simulink model "Supercap_Thermo_Electrical_Cell_Simulation_Model"  (R2024b)
settings: Solver=VariableStepAuto  StartTime=0.0  StopTime=Sim_TimeEnd_s
undefined symbols (not defined in the file): C, Cell_CapRated_F, Cell_HeatCapa_JpK, Cell_LowerSOCLimit_pc, Cell_LowerVoltageLimit_V, Cell_ResESR10ms_Ohm, Cell_ResESR1s_Ohm, Cell_RthToCooling_KpW, Cell_RthToEnvironment_KpW, Cell_TempInit_degC, Cell_UpperSOCLimit_pc, Cell_UpperVoltageLimit_V, Cell_VoltRated_V, Cell_VoltStart_V, Cooling_Temp_degC, Environment_Temp_degC, ESR, Sim_SocInit_pc, Sim_SOH_PU, Sim_TimeStep_s, Switch_CoolingONOFF, Switch_CurrentOrPower, Switch_DeratingONOFF_NN
libraries: simulink x11, slpidlib x1
settings Model: Creator=ludovico.barro  LastModifiedBy=francesco.bazzani
settings ModelReferenceCC: EnableRefExpFcnMdlSchedulingChecks=on
settings RTWCC: GPUComputeCapability=3.5

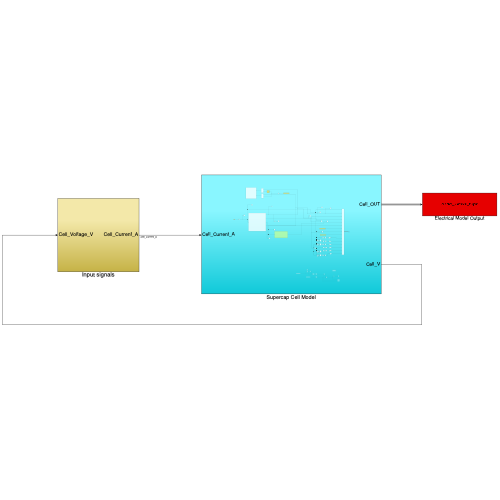
[thumbnail: Simulink's stored preview of the top-level diagram]
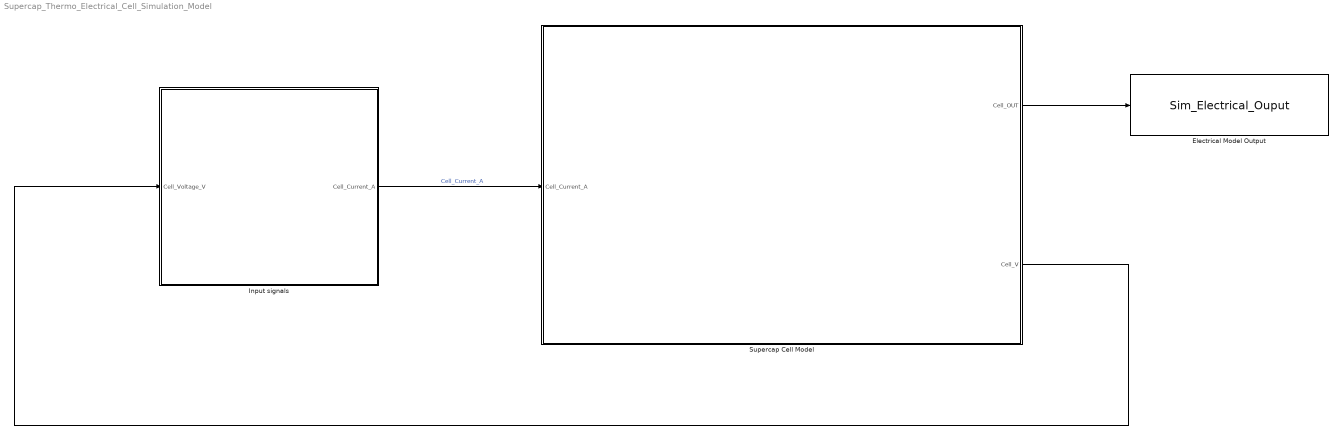
== system Supercap_Thermo_Electrical_Cell_Simulation_Model ==
  Electrical Model Output : ToWorkspace  VariableName=Sim_Electrical_Ouput  SaveFormat=Timeseries  SampleTime=Sim_TimeStep_s
  Input signals : Subsystem
  Supercap Cell Model : Subsystem
  wires:
  Supercap Cell Model/1(Cell_OUT) -> Electrical Model Output/1
  Input signals/1(Cell_Current_A) -> Supercap Cell Model/1(Cell_Current_A)  "Cell_Current_A"
  Supercap Cell Model/2(Cell_V) -> Input signals/1(Cell_Voltage_V)

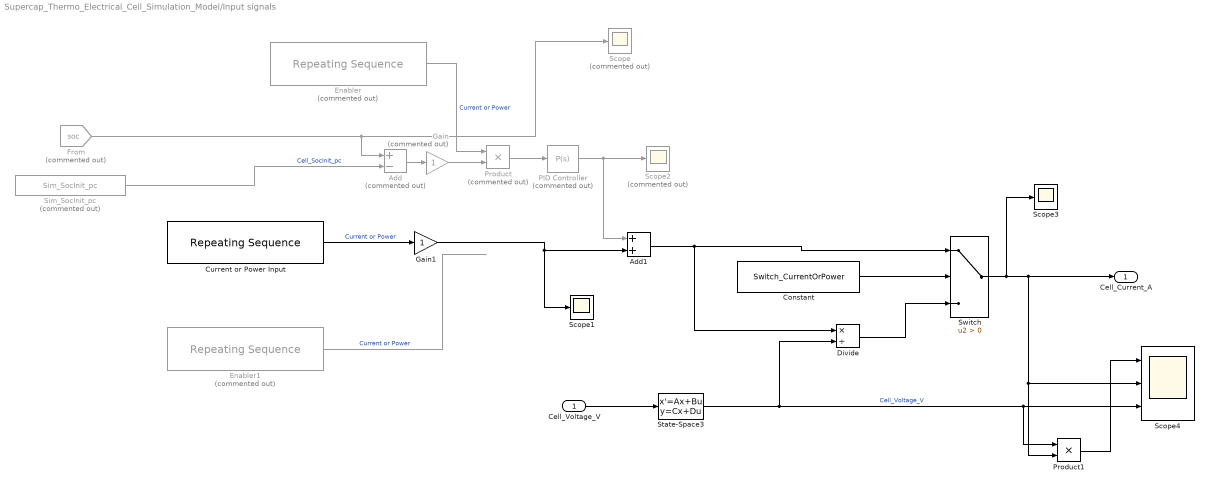
== system Supercap_Thermo_Electrical_Cell_Simulation_Model/Input signals ==
  Cell_Voltage_V : Inport
  Add : Sum  Commented=on  Inputs=+-
  Add1 : Sum
  Constant : Constant  Value=Switch_CurrentOrPower
  Current or Power Input : simulink/Sources/Repeating Sequence  rep_seq_t=Cell_LoadInputTime_s  rep_seq_y=Cell_LoadInputCurrOrPower_AW
  Divide : Product  Inputs=*/
  Enabler : simulink/Sources/Repeating Sequence  Commented=on  rep_seq_t=[0, 60,60.1, 20*60, 20*60+0.1]  rep_seq_y=[0,0,1,1,0]
  Enabler1 : simulink/Sources/Repeating Sequence  Commented=on  rep_seq_t=[0, 60,60.1, 20*60, 20*60+0.1]  rep_seq_y=[1,1,0,0,1]
  From : From  Commented=on  GotoTag=soc  TagVisibility=global
  Gain : Gain  Commented=on
  Gain1 : Gain
  PID Controller : slpidlib/PID Controller  Commented=on  Controller=P  Form=Parallel  TimeDomain=Continuous-time  UseExternalTs=off  SampleTime=-1  IntegratorMethod=Forward Euler  FilterMethod=Forward Euler  ControllerParametersSource=internal  P=1000  I=1  UseKiTs=off  D=0  UseExternalDerivativeSource=off  N=100  UseFilter=on  TunerSelectOption=Transfer Function Based (PID Tuner App)  InitialConditionSource=internal  InitialConditionForIntegrator=0  InitialConditionForFilter=0  DifferentiatorICPrevScaledInput=0  ExternalReset=none  TrackingMode=off  Kt=1  LimitOutput=on  SatLimitsSource=internal  UpperSaturationLimit=10  LowerSaturationLimit=-10  LinearizeAsGain=on  AntiWindupMode=none  Kb=1  LimitIntegrator=off  UpperIntegratorSaturationLimit=inf  LowerIntegratorSaturationLimit=-inf  POutMin=[]  POutMax=[]  IOutMin=[]  IOutMax=[]  DOutMin=[]  DOutMax=[]  NOutMin=[]  NOutMax=[]  SumOutMin=[]  SumOutMax=[]  SaturationOutMin=[]  SaturationOutMax=[]  PParamMin=[]  PParamMax=[]  IParamMin=[]  IParamMax=[]  DParamMin=[]  DParamMax=[]  NParamMin=[]  NParamMax=[]  KbParamMin=[]  KbParamMax=[]  KtParamMin=[]  KtParamMax=[]  KbOutMin=[]  KbOutMax=[]  KtOutMin=[]  KtOutMax=[]  IntegratorOutMin=[]  IntegratorOutMax=[]  FilterOutMin=[]  FilterOutMax=[]  SumI1OutMin=[]  SumI1OutMax=[]  SumI2OutMin=[]  SumI2OutMax=[]  SumI3OutMin=[]  SumI3OutMax=[]  SumI4OutMin=[]  SumI4OutMax=[]  SumDOutMin=[]  SumDOutMax=[]  DifferentiatorOutMin=[]  DifferentiatorOutMax=[]  FilterDiffOutCoefMin=[]  FilterDiffOutCoefMax=[]  ReciprocalOutMin=[]  ReciprocalOutMax=[]  SumDenOutMin=[]  SumDenOutMax=[]  SumNumOutMin=[]  SumNumOutMax=[]  DivideOutMin=[]  DivideOutMax=[]  UdiffTsProdOutMin=[]  UdiffTsProdOutMax=[]  NTsProdOutMin=[]  NTsProdOutMax=[]  UintegralTsProdOutMin=[]  UintegralTsProdOutMax=[]  UngainTsProdOutMin=[]  UngainTsProdOutMax=[]  ClampingZeroOutDataTypeStr=Inherit: Inherit via back propagation  ClampingZeroOutMin=[]  ClampingZeroOutMax=[]  FilterDenConstantOutDataTypeStr=Inherit: Inherit via back propagation  FilterDenConstantOutMin=[]  FilterDenConstantOutMax=[]  PCopyOutDataTypeStr=Inherit: Inherit via back propagation  PCopyOutMin=[]  PCopyOutMax=[]  NCopyOutDataTypeStr=Inherit: Inherit via back propagation  NCopyOutMin=[]  NCopyOutMax=[]  IntegratorContinuousStateAttributes=''  IntegratorStateMustResolveToSignalObject=off  IntegratorRTWStateStorageClass=Auto  FilterContinuousStateAttributes=''  FilterStateMustResolveToSignalObject=off  FilterRTWStateStorageClass=Auto  ParallelPVariant=InternalParameters  IdealPVariant=Disabled  IVariant=Disabled  DVariant=Disabled  IntegratorVariant=Disabled  SatVariant=Enabled  AWVariant=Disabled  PCopyVariant=Disabled  TRVariant=Disabled  FdbkBlocksVariant=Forward  IdealPFdbkVariant=Disabled  SatFdbkVariant=Disabled  DerivativeFilterVariant=Disabled  NVariant=Disabled  NCopyVariant=Disabled_SignalSpec  FilterICVariant=Disabled  IntegratorICVariant=Disabled  ExternalResetVariant=Disabled  TRSumVariant=Passthrough  SumFdbkVariant=Disabled  SumVariant=Passthrough_P  TsampFilterVariant=InternalTs  TsampNgainVariant=Passthrough  TsampIntegralVariant=Disabled_SignalSpec  ExternalSaturationOutDataTypeStr=Inherit: Same as second input  DerivativeSourceVariant=Disabled  PreIntVariant=InternalPreInt
  Product : Product  Commented=on
  Product1 : Product
  Scope : Scope  Commented=on
  Scope1 : Scope
  Scope2 : Scope  Commented=on
  Scope3 : Scope
  Scope4 : Scope  NumInputPorts=3
  Sim_SocInit_pc : Constant  Commented=on  Value=Sim_SocInit_pc
  State-Space3 : StateSpace  A=-1/1e-6  B=1/1e-6  D=0  InitialCondition=Cell_VoltStart_V
  Switch : Switch  Criteria=u2 > Threshold  SaturateOnIntegerOverflow=off  InputSameDT=off
  Cell_Current_A : Outport
  wires:
  Constant/1 -> Switch/2
  Switch/1 -> Scope3/1, Scope4/2, Product1/2, Cell_Current_A/1
  Cell_Voltage_V/1 -> State-Space3/1
  State-Space3/1 -> Product1/1, Scope4/3, Divide/2  "Cell_Voltage_V"
  Divide/1 -> Switch/3
  Sim_SocInit_pc/1 -> Add/2  "Cell_SocInit_pc"
  From/1 -> Add/1, Scope/1
  Add/1 -> Gain/1
  Product/1 -> PID Controller/1
  Enabler/1 -> Product/1  "Current or Power"
  PID Controller/1 -> Scope2/1, Add1/1
  Add1/1 -> Divide/1, Switch/1
  Current or Power Input/1 -> Gain1/1  "Current or Power"
  Gain1/1 -> Scope1/1, Add1/2
  Enabler1/1 -> ?  "Current or Power"
  Gain/1 -> Product/2
  Product1/1 -> Scope4/1

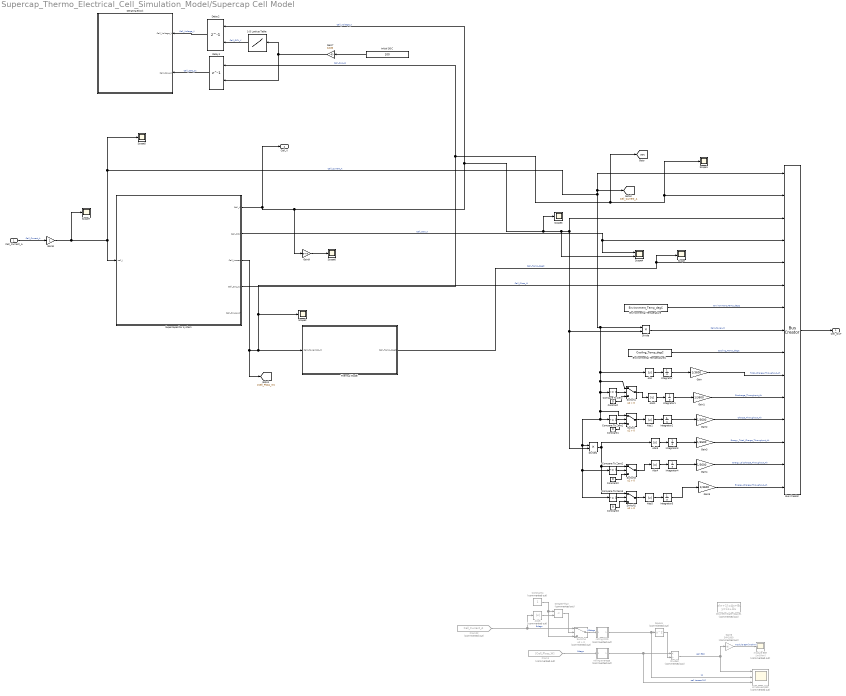
== system Supercap_Thermo_Electrical_Cell_Simulation_Model/Supercap Cell Model ==
  Cell_Current_A : Inport
  1-D Lookup Table : Lookup_n-D  NumberOfTableDimensions=1  BreakpointsForDimension1=linspace(0,1,1000)  Table=linspace(0,1,1000).^(1/2)*3  InternalRulePriority=Speed  RndMeth=Simplest
  Abs{,1..5} (6 alike) : Abs  SaturateOnIntegerOverflow=off
  Abs6 : Abs  Commented=on  SaturateOnIntegerOverflow=off
  Bus Creator : BusCreator  Inputs=15
  Compare To Zero : simulink/Logic and Bit Operations/Compare To Zero  relop=<=  OutDataTypeStr=boolean
  Compare To Zero1 : simulink/Logic and Bit Operations/Compare To Zero  relop=>=  OutDataTypeStr=boolean
  Compare To Zero2 : simulink/Logic and Bit Operations/Compare To Zero  relop=<=  OutDataTypeStr=boolean
  Compare To Zero3 : simulink/Logic and Bit Operations/Compare To Zero  relop=>=  OutDataTypeStr=boolean
  Constant{,1..3} (4 alike) : Constant  Value=0
  Constant4 : Constant  Commented=on
  Delay1 : Delay  DelayLength=1  InitialConditionSource=Input port
      settings: InputPortMap=u0,p4
  Delay2 : Delay  DelayLength=1  InitialConditionSource=Input port
      settings: InputPortMap=u0,p4
  Derating Block : Subsystem
  Discrete State-Space1 : DiscreteStateSpace  Commented=on  A=-1/(1e-6)  B=1/(1e-6)  D=0  SampleTime=-1
  Divide : Product  Inputs=**
  Divide1 : Product  Inputs=**
  Divide2 : Product  Commented=on  Inputs=*/
  Environmental Temperature : Constant  Value=Environment_Temp_degC
  Environmental Temperature1 : Constant  Value=Cooling_Temp_degC
  From1 : From  Commented=on  GotoTag=Cell_Ploss_W
  From22 : From  Commented=on  GotoTag=Cell_Current_A  TagVisibility=global
  Gain{,1..5} (6 alike) : Gain  Gain=1/3600
  Gain6 : Gain  Commented=on  Gain=54*1000
  Gain7 : Gain  Gain=1/100
  Gain8 : Gain
  Gain9 : Gain  Gain=54*9
  GreaterThan : RelationalOperator  Commented=on  Operator=<  OutDataTypeStr=boolean  RndMeth=Simplest  InputSameDT=off
  Initial SOC : Constant  Value=100
  Integrator{,1..5} (6 alike) : Integrator
  Scope{,1..3,5..7} (7 alike) : Scope
  Scope4 : Scope  NumInputPorts=2
  Square : Math  Commented=on  Operator=square
  Supercapacitor system : Subsystem  mask{Cell_ResESR10ms_Ohm=Cell_ResESR10ms_Ohm, Cell_ResESR1s_Ohm=Cell_ResESR1s_Ohm, Cell_CapRated_F=Cell_CapRated_F, Cell_VoltRated_V=Cell_VoltRated_V, Cell_SoCInit_PU=Sim_SocInit_pc, Cell_SOH_PU=Sim_SOH_PU, cell_count=54, add_Res=1.12, bridge_Res=0.8}
      mask prompts: Cell_ResESR10ms_Ohm "Rated 10ms ESR [Ohm]"; Cell_ResESR1s_Ohm "Rated 1s ESR [Ohm]"; Cell_CapRated_F "Rated Capacitance [F]"; Cell_VoltRated_V "Rated V [V]"; Cell_SoCInit_PU "SoC [PU]"; Cell_SOH_PU "SoH [PU]"; cell_count "cells per module"; add_Res "Additional module R"; bridge_Res "Bridge R"
      mask DialogControl Container6 Prompt: Cell
      mask DialogControl Container4 Prompt: Module
      mask Display: image('Skeleton-SCX5000-300x300.jpg');
  Switch{,1..3} (4 alike) : Switch  Criteria=u2 > Threshold  SaturateOnIntegerOverflow=off  InputSameDT=off
  Switch4 : Switch  Commented=on  Criteria=u2 > Threshold  SaturateOnIntegerOverflow=off  InputSameDT=off
  Thermal Model : Subsystem
      mask Display: image('fluid_flow.png'); % Use "Edit Image" on toolstrip to change.
  Windowed ESR : Scope  Commented=on  NumInputPorts=3
  module ESR [mOhm] : Scope  Commented=on
  rolling RMS : Subsystem  Commented=on  mask{t_window=60}
      mask prompts: t_window "window time [s]"
  rolling average : Subsystem  Commented=on  mask{t_window=60}
      mask prompts: t_window "window time [s]"
  Cell_OUT : Outport
  Cell_V : Outport  Port=2
  tag scope: Cell_Current_A=global, soc=global
  wires:
  Thermal Model/1(Cell_Temp_degC) -> Scope/1, Bus Creator/5  "Cell_Temp_degC"
  Supercapacitor system/3(Cell_Losses) -> Thermal Model/1(Cell_Powerloss_W), Scope2/1, Bus Creator/6, [Cell_Ploss_W]  "Cell_Ploss_W"
  Supercapacitor system/4(Cell_Soc_pu) -> Delay1/1, [soc], Scope1/1, Bus Creator/2  "Cell_Soc_pc"
  Environmental Temperature/1 -> Bus Creator/7  "Environment_Temp_degC"
  Supercapacitor system/1(Cell_V) -> Cell_V/1, Gain9/1, Delay2/1, Scope3/1, Scope4/2, Bus Creator/3, Divide1/2, Divide/2  "Cell_Voltage_V"
  Supercapacitor system/2(Cell_OCV) -> Scope4/1, Bus Creator/4  "Cell_OCV_V"
  Bus Creator/1 -> Cell_OUT/1
  Divide/1 -> Bus Creator/8  "Cell_Power_W"
  Environmental Temperature1/1 -> Bus Creator/9  "Cooling_Temp_degC"
  Delay1/1 -> Derating Block/2(Cell_Soc_pc)  "Cell_SOC_pc"
  1-D Lookup Table/1 -> Delay2/2  "Cell_OCV_V"
  Delay2/1 -> Derating Block/1(Cell_Voltage_V)  "Cell_Voltage_V"
  Initial SOC/1 -> Gain7/1
  Integrator/1 -> Gain/1
  Abs/1 -> Integrator/1
  Gain/1 -> Bus Creator/10  "Total_Charge_Throughput_Ah"
  Gain1/1 -> Bus Creator/11  "Discharge_Throughput_Ah"
  Switch1/1 -> Abs1/1
  Integrator1/1 -> Gain1/1
  Integrator2/1 -> Gain2/1
  Switch/1 -> Abs2/1
  Gain2/1 -> Bus Creator/12  "Charge_Throughput_Ah"
  Abs1/1 -> Integrator1/1
  Abs2/1 -> Integrator2/1
  Compare To Zero/1 -> Switch1/2
  Constant/1 -> Switch1/3
  Constant1/1 -> Switch/3
  Compare To Zero1/1 -> Switch/2
  Compare To Zero3/1 -> Switch2/2
  Constant3/1 -> Switch2/3
  Constant2/1 -> Switch3/3
  Compare To Zero2/1 -> Switch3/2
  Abs5/1 -> Integrator5/1
  Abs4/1 -> Integrator4/1
  Gain5/1 -> Bus Creator/15  "Energy_Charge_Throughput_Ah"
  Switch2/1 -> Abs5/1
  Integrator5/1 -> Gain5/1
  Cell_Current_A/1 -> Gain8/1  "Cell_Current_A"
  Integrator4/1 -> Gain4/1
  Switch3/1 -> Abs4/1
  Gain4/1 -> Bus Creator/14  "Energy_Discharge_Throughput_Ah"
  Gain3/1 -> Bus Creator/13  "Energy_Total_Charge_Throughput_Ah"
  Abs3/1 -> Integrator3/1
  Integrator3/1 -> Gain3/1
  Divide1/1 -> Abs3/1, Switch2/1, Switch3/1
  Constant4/1 -> Switch4/3, GreaterThan/1
  rolling average/1(Out1) -> Divide2/1, Windowed ESR/3  "cell Losses [W]"
  Switch4/1 -> rolling RMS/1(In1)  "55degc"
  Gain6/1 -> module ESR [mOhm]/1  "module ESR [mOhm]"
  Abs6/1 -> GreaterThan/2
  Square/1 -> Divide2/2
  Divide2/1 -> Windowed ESR/1, Gain6/1  "cell ESR"
  rolling RMS/1(Out1) -> Windowed ESR/2, Square/1  "1s"
  From22/1 -> Switch4/1, Abs6/1  "5degc"
  GreaterThan/1 -> Switch4/2
  From1/1 -> rolling average/1(In1)  "5degc"
  Gain7/1 -> Delay1/2, 1-D Lookup Table/1
  Gain8/1 -> Scope7/1, Scope5/1, [Cell_Current_A], Bus Creator/1, Compare To Zero1/1, Compare To Zero3/1, Compare To Zero2/1, Divide1/1, Switch/1, Compare To Zero/1, Switch1/1, Abs/1, Divide/1, Supercapacitor system/1(cell_I)  "Cell_Current_A"
  Gain9/1 -> Scope6/1

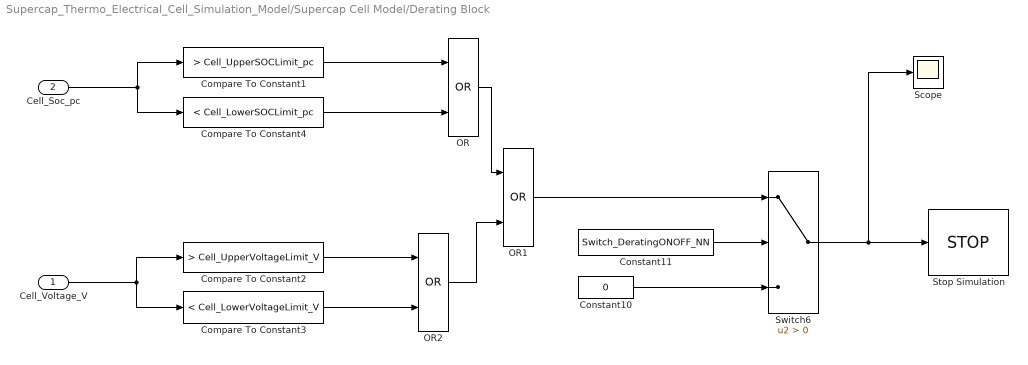
== system Supercap_Thermo_Electrical_Cell_Simulation_Model/Supercap Cell Model/Derating Block ==
  Cell_Voltage_V : Inport
  Cell_Soc_pc : Inport  Port=2
  Compare To Constant1 : simulink/Logic and Bit Operations/Compare To Constant  relop=>  const=Cell_UpperSOCLimit_pc  OutDataTypeStr=boolean
  Compare To Constant2 : simulink/Logic and Bit Operations/Compare To Constant  relop=>  const=Cell_UpperVoltageLimit_V  OutDataTypeStr=boolean
  Compare To Constant3 : simulink/Logic and Bit Operations/Compare To Constant  relop=<  const=Cell_LowerVoltageLimit_V  OutDataTypeStr=boolean
  Compare To Constant4 : simulink/Logic and Bit Operations/Compare To Constant  relop=<  const=Cell_LowerSOCLimit_pc  OutDataTypeStr=boolean
  Constant10 : Constant  Value=0
  Constant11 : Constant  Value=Switch_DeratingONOFF_NN
  OR : Logic  Operator=OR  IconShape=distinctive  AllPortsSameDT=off  OutDataTypeStr=boolean
  OR1 : Logic  Operator=OR  IconShape=distinctive  AllPortsSameDT=off  OutDataTypeStr=boolean
  OR2 : Logic  Operator=OR  IconShape=distinctive  AllPortsSameDT=off  OutDataTypeStr=boolean
  Scope : Scope
  Stop Simulation : Stop
  Switch6 : Switch  Criteria=u2 > Threshold  SaturateOnIntegerOverflow=off  InputSameDT=off
  wires:
  Cell_Soc_pc/1 -> Compare To Constant1/1, Compare To Constant4/1
  Compare To Constant4/1 -> OR/2
  Compare To Constant1/1 -> OR/1
  Cell_Voltage_V/1 -> Compare To Constant3/1, Compare To Constant2/1
  OR/1 -> OR1/1
  OR2/1 -> OR1/2
  OR1/1 -> Switch6/1
  Switch6/1 -> Scope/1, Stop Simulation/1
  Constant11/1 -> Switch6/2
  Constant10/1 -> Switch6/3
  Compare To Constant2/1 -> OR2/1
  Compare To Constant3/1 -> OR2/2

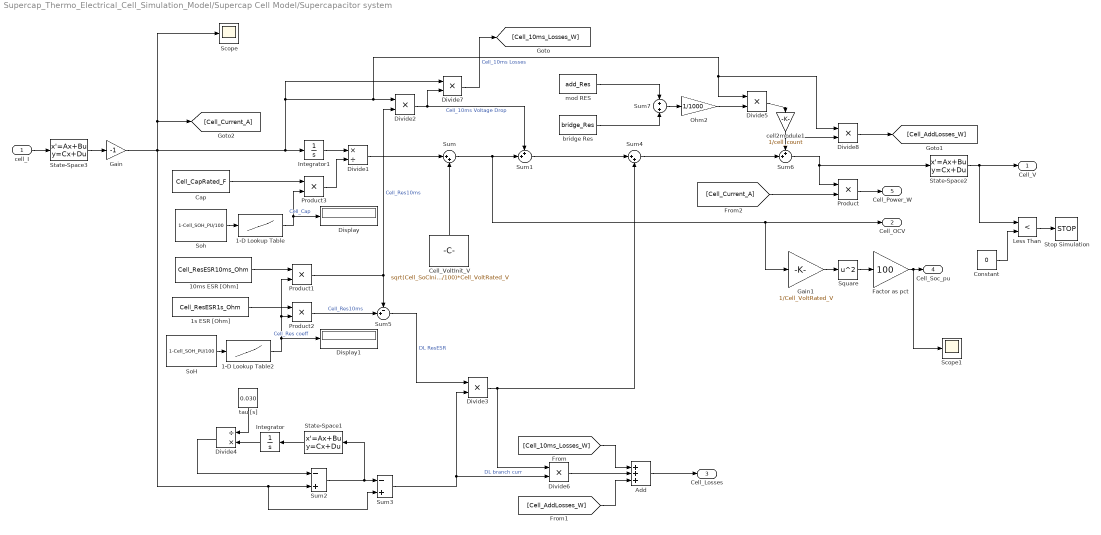
== system Supercap_Thermo_Electrical_Cell_Simulation_Model/Supercap Cell Model/Supercapacitor system ==
  cell_I : Inport
  1-D Lookup Table : Lookup_n-D  NumberOfTableDimensions=1  BreakpointsForDimension1=C(:,1)  Table=C(:,2)  InternalRulePriority=Speed  RndMeth=Simplest
  1-D Lookup Table2 : Lookup_n-D  NumberOfTableDimensions=1  BreakpointsForDimension1=ESR(:,1)  Table=ESR(:,2)  InternalRulePriority=Speed  RndMeth=Simplest
  10ms ESR [Ohm] : Constant  Value=Cell_ResESR10ms_Ohm
  1s ESR [Ohm] : Constant  Value=Cell_ResESR1s_Ohm
  Add : Sum  Inputs=+++
  Cap : Constant  Value=Cell_CapRated_F
  Cell_VoltInit_V : Constant  Value=sqrt(Cell_SoCInit_PU/100)*Cell_VoltRated_V
  Constant : Constant  Value=0
  Display : Display
  Display1 : Display
  Divide1 : Product  Inputs=*/
  Divide{2..3,5..8} (6 alike) : Product  Inputs=**
  Divide4 : Product  Inputs=/*
  Factor as pct : Gain  Gain=100
  Gain : Gain  Gain=-1
  Gain1 : Gain  Gain=1/Cell_VoltRated_V
  Integrator : Integrator
  Integrator1 : Integrator
  Less Than : RelationalOperator  Operator=<  OutDataTypeStr=boolean  RndMeth=Simplest  InputSameDT=off
  Ohm2 : Gain  Gain=1/1000
  Product{,1..3} (4 alike) : Product
  Scope : Scope
  Scope1 : Scope
  SoH : Constant  Value=1-Cell_SOH_PU/100
  Soh : Constant  Value=1-Cell_SOH_PU/100
  Square : Math  Operator=square
  State-Space1 : StateSpace  A=-1/1e-6  B=1/1e-6  D=0  InitialCondition=0
  State-Space2 : StateSpace  A=-1/1e-6  B=1/1e-6  D=0  InitialCondition=sqrt(Cell_SoCInit_PU/100)*Cell_VoltRated_V
  State-Space3 : StateSpace  A=-1/1e-6  B=1/1e-6  D=0  InitialCondition=0
  Stop Simulation : Stop
  Sum : Sum  Inputs=|++
  Sum1 : Sum  Inputs=++|
  Sum2 : Sum  Inputs=-+
  Sum3 : Sum  Inputs=-+
  Sum4 : Sum  Inputs=|++
  Sum5 : Sum  Inputs=-+|
  Sum6 : Sum  Inputs=++|
  Sum7 : Sum  Inputs=+|+
  bridge Res : Constant  Value=bridge_Res
  cell2module1 : Gain  Gain=1/cell_count
  mod RES : Constant  Value=add_Res
  tau [s] : Constant  Value=0.030
  Cell_V : Outport
  Cell_OCV : Outport  Port=2
  Cell_Losses : Outport  Port=3
  Cell_Soc_pu : Outport  Port=4
  Cell_Power_W : Outport  Port=5
  wires:
  Cell_VoltInit_V/1 -> Sum/2
  Integrator1/1 -> Divide1/1
  Product1/1 -> Sum5/1, Divide2/2  "Cell_Res10ms"
  Divide2/1 -> Divide7/2, Sum1/1  "Cell_10ms Voltage Drop"
  tau [s]/1 -> Divide4/1
  Divide3/1 -> Sum4/2, Divide6/1
  Sum1/1 -> Sum4/1
  Divide4/1 -> Sum2/1
  Divide1/1 -> Sum/1
  Sum2/1 -> Sum3/1, State-Space1/1
  Sum5/1 -> Divide3/1  "DL ResESR"
  Integrator/1 -> Divide4/2
  Sum3/1 -> Divide3/2, Divide6/2  "DL branch curr"
  cell_I/1 -> State-Space3/1
  Sum4/1 -> Sum6/2
  Sum6/1 -> Product/1, State-Space2/1
  Divide5/1 -> cell2module1/1
  mod RES/1 -> Sum7/1
  Ohm2/1 -> Divide5/2
  Sum7/1 -> Ohm2/1
  bridge Res/1 -> Sum7/2
  cell2module1/1 -> Sum6/1, Divide8/2
  Gain/1 -> Scope/1, [Cell_Current_A], Integrator1/1, Divide7/1, Divide8/1, Divide5/1, Divide2/1, Sum3/2, Sum2/2
  Divide6/1 -> Add/2
  Divide7/1 -> [Cell_10ms_Losses_W]  "Cell_10ms Losses"
  [Cell_10ms_Losses_W] -> Add/1
  Add/1 -> Cell_Losses/1
  Divide8/1 -> [Cell_AddLosses_W]
  [Cell_AddLosses_W] -> Add/3
  Gain1/1 -> Square/1
  Square/1 -> Factor as pct/1
  [Cell_Current_A] -> Product/2
  Product/1 -> Cell_Power_W/1
  Sum/1 -> Gain1/1, Cell_OCV/1, Sum1/2
  State-Space1/1 -> Integrator/1
  State-Space2/1 -> Less Than/1, Cell_V/1
  State-Space3/1 -> Gain/1
  Factor as pct/1 -> Scope1/1, Cell_Soc_pu/1
  Constant/1 -> Less Than/2
  Less Than/1 -> Stop Simulation/1
  SoH/1 -> 1-D Lookup Table2/1
  10ms ESR [Ohm]/1 -> Product1/1
  1-D Lookup Table2/1 -> Display1/1, Product2/2, Product1/2  "Cell_Res coeff"
  1s ESR [Ohm]/1 -> Product2/1
  Product2/1 -> Sum5/2  "Cell_Res10ms"
  Soh/1 -> 1-D Lookup Table/1
  1-D Lookup Table/1 -> Display/1, Product3/2  "Cell_Cap"
  Cap/1 -> Product3/1
  Product3/1 -> Divide1/2

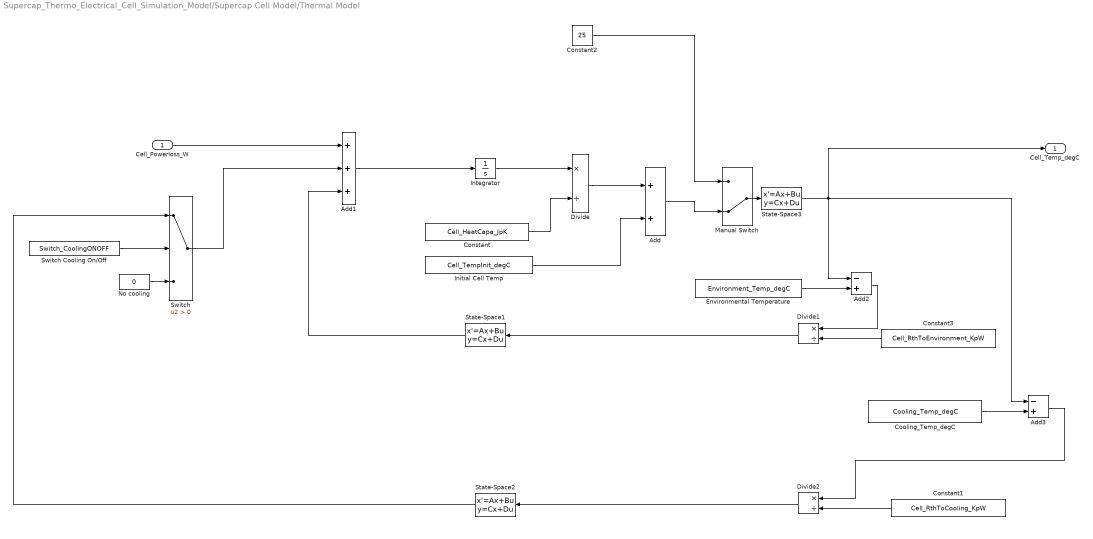
== system Supercap_Thermo_Electrical_Cell_Simulation_Model/Supercap Cell Model/Thermal Model ==
  Cell_Powerloss_W : Inport
  Add : Sum
  Add1 : Sum  Inputs=+++
  Add2 : Sum  Inputs=-+
  Add3 : Sum  Inputs=-+
  Constant : Constant  Value=Cell_HeatCapa_JpK
  Constant1 : Constant  Value=Cell_RthToCooling_KpW
  Constant2 : Constant  Value=25
  Constant3 : Constant  Value=Cell_RthToEnvironment_KpW
  Cooling_Temp_degC : Constant  Value=Cooling_Temp_degC
  Divide : Product  Inputs=*/
  Divide1 : Product  Inputs=*/
  Divide2 : Product  Inputs=*/
  Environmental Temperature : Constant  Value=Environment_Temp_degC
  Initial Cell Temp : Constant  Value=Cell_TempInit_degC
  Integrator : Integrator
  Manual Switch : ManualSwitch  CurrentSetting=0
  No cooling : Constant  Value=0
  State-Space1 : StateSpace  A=-1/1e-6  B=1/1e-6  D=0  InitialCondition=0
  State-Space2 : StateSpace  A=-1/1e-6  B=1/1e-6  D=0  InitialCondition=0
  State-Space3 : StateSpace  A=-1/1e-6  B=1/1e-6  D=0  InitialCondition=Environment_Temp_degC
  Switch : Switch  Criteria=u2 > Threshold  SaturateOnIntegerOverflow=off  InputSameDT=off
  Switch Cooling On/Off : Constant  Value=Switch_CoolingONOFF
  Cell_Temp_degC : Outport
  wires:
  Constant3/1 -> Divide1/2
  Add2/1 -> Divide1/1
  Divide1/1 -> State-Space1/1
  Constant/1 -> Divide/2
  Divide/1 -> Add/1
  Add1/1 -> Integrator/1
  State-Space1/1 -> Add1/3
  Integrator/1 -> Divide/1
  Environmental Temperature/1 -> Add2/2
  Initial Cell Temp/1 -> Add/2
  Cell_Powerloss_W/1 -> Add1/1
  Manual Switch/1 -> State-Space3/1
  Cooling_Temp_degC/1 -> Add3/2
  Add3/1 -> Divide2/1
  State-Space2/1 -> Switch/1
  Constant1/1 -> Divide2/2
  Divide2/1 -> State-Space2/1
  Switch/1 -> Add1/2
  No cooling/1 -> Switch/3
  Switch Cooling On/Off/1 -> Switch/2
  Constant2/1 -> Manual Switch/1
  Add/1 -> Manual Switch/2
  State-Space3/1 -> Cell_Temp_degC/1, Add2/1, Add3/1

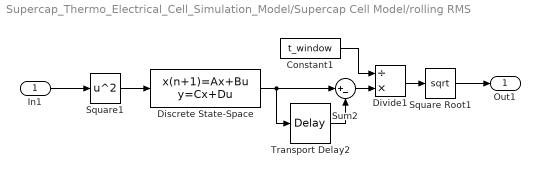
== system Supercap_Thermo_Electrical_Cell_Simulation_Model/Supercap Cell Model/rolling RMS ==
  In1 : Inport
  Constant1 : Constant  Value=t_window
  Discrete State-Space : DiscreteStateSpace  A=0  D=0  SampleTime=-1
  Divide1 : Product  Inputs=/*
  Square Root1 : Sqrt
  Square1 : Math  Operator=square
  Sum2 : Sum  Inputs=|+-
  Transport Delay2 : TransportDelay  DelayTime=t_window
  Out1 : Outport
  wires:
  Divide1/1 -> Square Root1/1
  Sum2/1 -> Divide1/2
  Constant1/1 -> Divide1/1
  In1/1 -> Square1/1
  Discrete State-Space/1 -> Transport Delay2/1, Sum2/1
  Transport Delay2/1 -> Sum2/2
  Square Root1/1 -> Out1/1
  Square1/1 -> Discrete State-Space/1

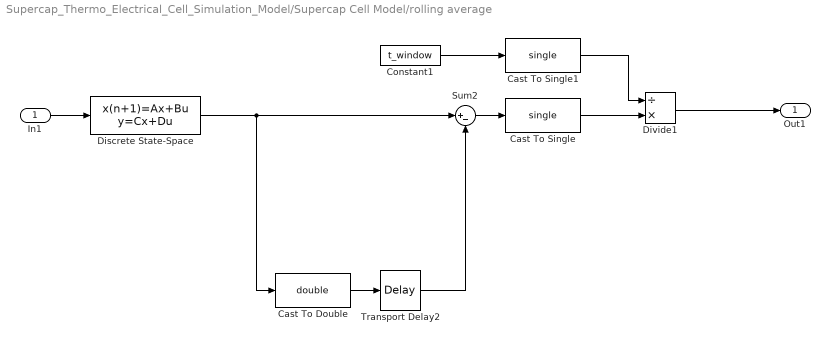
== system Supercap_Thermo_Electrical_Cell_Simulation_Model/Supercap Cell Model/rolling average ==
  In1 : Inport
  Cast To Double : DataTypeConversion  OutDataTypeStr=double  SaturateOnIntegerOverflow=off  RndMeth=Floor
  Cast To Single : DataTypeConversion  OutDataTypeStr=single  SaturateOnIntegerOverflow=off  RndMeth=Floor
  Cast To Single1 : DataTypeConversion  OutDataTypeStr=single  SaturateOnIntegerOverflow=off  RndMeth=Floor
  Constant1 : Constant  Value=t_window
  Discrete State-Space : DiscreteStateSpace  A=0  D=0  SampleTime=-1
  Divide1 : Product  Inputs=/*
  Sum2 : Sum  Inputs=|+-
  Transport Delay2 : TransportDelay  DelayTime=t_window
  Out1 : Outport
  wires:
  Sum2/1 -> Cast To Single/1
  Constant1/1 -> Cast To Single1/1
  Discrete State-Space/1 -> Sum2/1, Cast To Double/1
  Transport Delay2/1 -> Sum2/2
  Divide1/1 -> Out1/1
  In1/1 -> Discrete State-Space/1
  Cast To Double/1 -> Transport Delay2/1
  Cast To Single/1 -> Divide1/2
  Cast To Single1/1 -> Divide1/1
